simulink model "student_control"  (Simulink 8.0)
settings: Solver=FixedStepDiscrete  StartTime=0.0  StopTime=10.0  FixedStep=SampleTime  RelTol=1e-3
libraries: simulink x1
settings Model: Creator=austinmurch  LastModifiedBy=brtaylor
settings DataIOCC: SignalLoggingSaveFormat=ModelDataLogs
settings OptimizationCC: InlineParams=on  SimCompilerOptimization=On
settings DebuggingCC: FcnCallInpInsideContextMsg=UseLocalSettings  StrictBusMsg=Warning
settings HardwareCC: ProdLargestAtomicInteger=Long  ProdLargestAtomicFloat=Double  ProdIntDivRoundTo=Zero  ProdEndianess=BigEndian  ProdHWDeviceType=Freescale->32-bit PowerPC
settings ModelReferenceCC: ModelReferenceNumInstancesAllowed=Single
settings RTWCC: GenCodeOnly=on  GenerateMakefile=off  GenerateReport=on  CustomSourceCode="#include \"../../../Software/FlightCode/control/rtw_grt_control.c\""  LaunchReport=on
settings GRTTargetCC: CombineOutputUpdateFcns=off  GRTInterface=on

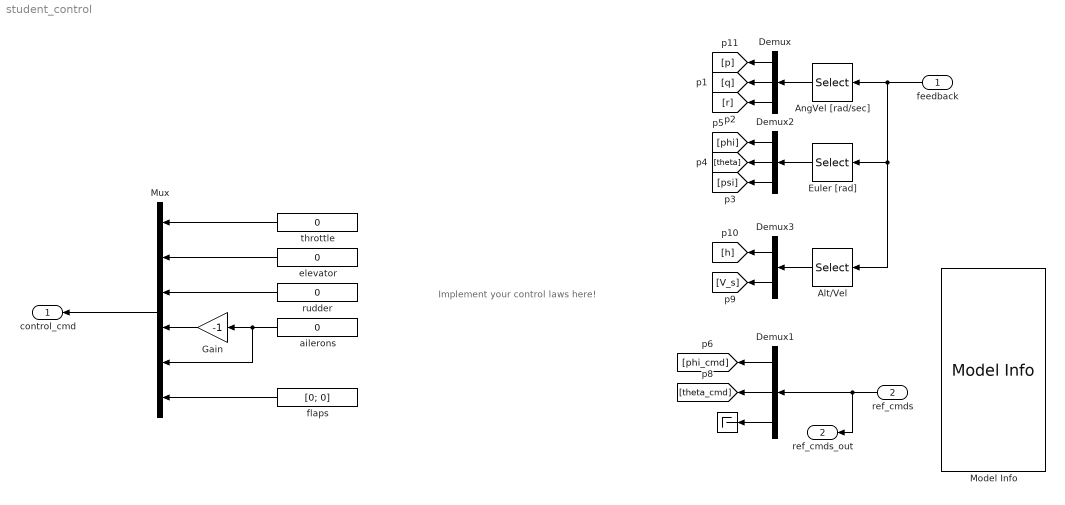
== system student_control ==
  note: Implement your control
      | laws here!
  feedback : Inport
  ref_cmds : Inport  Port=2
  " " : Terminator
  Alt/Vel : Selector  InputPortWidth=19  IndexOptions=Index vector (dialog)  Indices=[10:11]  OutputSizes=1
  AngVel [rad/sec] : Selector  InputPortWidth=19  IndexOptions=Index vector (dialog)  Indices=[4:6]  OutputSizes=1
  Demux : Demux  Outputs=3
  Demux1 : Demux  Outputs=[1 1 10]
  Demux2 : Demux  Outputs=3
  Demux3 : Demux  Outputs=2
  Euler [rad] : Selector  InputPortWidth=19  IndexOptions=Index vector (dialog)  Indices=[1:3]  OutputSizes=1
  Gain : Gain  Gain=-1
  Model Info : simulink/Model-Wide Utilities/Model Info  InitialBlockCM=None  BlockCM=None  Frame=on  DisplayStringWithTags=|  HorizontalTextAlignment=Center  LeftAlignmentValue=0.5  SourceBlockDiagram=student_control  TagMaxNumber=20
      | Ref Cmd Port Info
      | 
      | 1. phi_cmd
      | 2. theta_cmd
      | 3. psi_cmd
      | 4. p_cmd
      | 5. q_cmd
      | 6. r_cmd
      | 7. V_s_cmd
      | 8. h_cmd
      | 9. gndtrk_cmd
      | 10. aoa_cmd
      | 11. aos_cmd
      | 12. gamma_cmd
  Mux : Mux  Inputs=6
  ailerons : Constant  Value=0
  elevator : Constant  Value=0
  flaps : Constant  Value=[0; 0]
  rudder : Constant  Value=0
  throttle : Constant  Value=0
  control_cmd : Outport
  ref_cmds_out : Outport  Port=2
  wires:
  AngVel [rad/sec]/1 -> Demux/1
  Euler [rad]/1 -> Demux2/1
  Demux/1 -> [p]
  Demux/2 -> [q]
  Demux/3 -> [r]
  Demux2/3 -> [psi]
  feedback/1 -> AngVel [rad/sec]/1, Euler [rad]/1, Alt/Vel/1
  Mux/1 -> control_cmd/1
  flaps/1 -> Mux/6
  Demux2/2 -> [theta]
  Demux2/1 -> [phi]
  Alt/Vel/1 -> Demux3/1
  Demux3/2 -> [V_s]
  Demux3/1 -> [h]
  Gain/1 -> Mux/4
  throttle/1 -> Mux/1
  elevator/1 -> Mux/2
  rudder/1 -> Mux/3
  ailerons/1 -> Gain/1, Mux/5
  Demux1/1 -> [phi_cmd]
  Demux1/2 -> [theta_cmd]
  Demux1/3 -> " "/1
  ref_cmds/1 -> Demux1/1, ref_cmds_out/1
